simulink model "model_V2slx"  (R2024b)
settings: Solver=VariableStepAuto  StartTime=0.0  StopTime=30  RelTol=1e-3
values from neighbouring files (symbols this model uses):
  L = Simulink.Parameter    [initialization.m]    (also in mpc_v2.m = 0.35)
  Ts = 0.02    [mpc_v2.m]
libraries: simulink_extras x3, drivingscenarioandsensors x2, mpclib x1, robotmobilelib x1
settings Model: Creator=zanhe  LastModifiedBy=zanhe
settings OptimizationCC: DefaultParameterBehavior=Inlined  UseDivisionForNetSlopeComputation=on  GainParamInheritBuiltInType=on  UseFloatMulNetSlope=on  InlineInvariantSignals=on  PassReuseOutputArgsAs=Individual arguments  ZeroExternalMemoryAtStartup=off  ZeroInternalMemoryAtStartup=off  NoFixptDivByZeroProtection=on  EfficientFloat2IntCast=on  LifeSpan=1  OptimizeBlockOrder=speed  DifferentSizesBufferReuse=on  EfficientTunableParamExpr=on
settings DebuggingCC: ParameterTunabilityLossMsg=error  UniqueDataStoreMsg=error
settings HardwareCC: ProdBitPerPointer=32  ProdBitPerSizeT=32  ProdBitPerPtrDiffT=32  ProdLargestAtomicInteger=Long  ProdLargestAtomicFloat=Double  ProdWordSize=32  ProdLongLongMode=on  ProdHWDeviceType=ARM Compatible->ARM Cortex-M
settings SFSimCC: MATLABDynamicMemAlloc=off
settings RTWCC: Description=Embedded Coder  SystemTargetFile=ert.tlc  TemplateMakefile=ert_default_tmf
settings CodeAppCC: ForceParamTrailComments=on  IgnoreCustomStorageClasses=off  OperatorAnnotations=on  SimulinkDataObjDesc=on  SFDataObjDesc=on  CustomSymbolStrGlobalVar=rt$N$M  CustomSymbolStrType=$N$M  CustomSymbolStrFcn=$N$M$F  CustomSymbolStrMacro=$N$M  InsertBlockDesc=on
settings ERTTargetCC: TargetLangStandard=C99 (ISO)  GenerateSampleERTMain=on  IncludeMdlTerminateFcn=off  CombineSignalStateStructs=on  SupportAbsoluteTime=off  SupportComplex=off  SupportNonInlinedSFcns=on  ERTCustomFileTemplate=example_file_process.tlc  ERTFilePackagingFormat=CompactWithDataFile

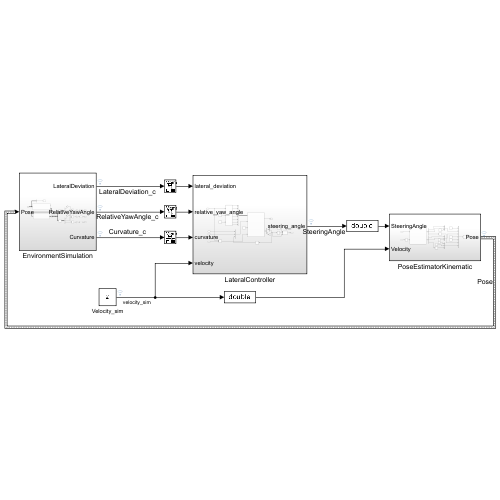
[thumbnail: Simulink's stored preview of the top-level diagram]
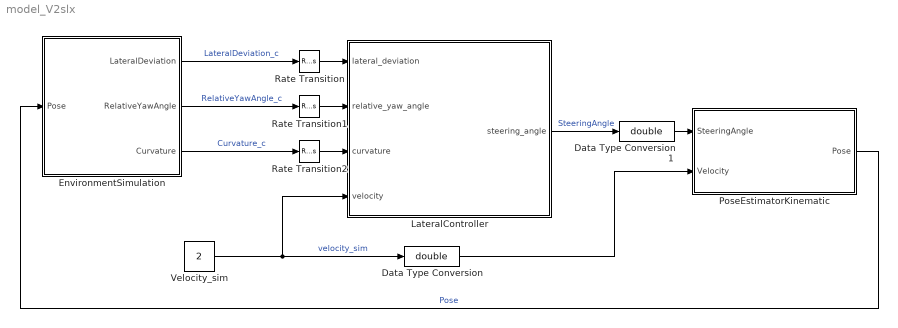
== system model_V2slx ==
  Data Type Conversion : DataTypeConversion  OutDataTypeStr=double  SaturateOnIntegerOverflow=off  RndMeth=Floor
  Data Type Conversion1 : DataTypeConversion  OutDataTypeStr=double  SaturateOnIntegerOverflow=off  RndMeth=Floor
  EnvironmentSimulation : Subsystem
  LateralController : Subsystem
  PoseEstimatorKinematic : Subsystem
  Rate Transition : RateTransition  Deterministic=off  OutPortSampleTime=Ts
  Rate Transition1 : RateTransition  Deterministic=off  OutPortSampleTime=Ts
  Rate Transition2 : RateTransition  Deterministic=off  OutPortSampleTime=Ts
  Velocity_sim : Constant  Value=2  OutDataTypeStr=single
  wires:
  Rate Transition/1 -> LateralController/1(lateral_deviation)
  Data Type Conversion1/1 -> PoseEstimatorKinematic/1(SteeringAngle)
  EnvironmentSimulation/3(Curvature) -> Rate Transition2/1  "Curvature_c"
  Rate Transition1/1 -> LateralController/2(relative_yaw_angle)
  Rate Transition2/1 -> LateralController/3(curvature)
  Velocity_sim/1 -> LateralController/4(velocity), Data Type Conversion/1  "velocity_sim"
  EnvironmentSimulation/2(RelativeYawAngle) -> Rate Transition1/1  "RelativeYawAngle_c"
  Data Type Conversion/1 -> PoseEstimatorKinematic/2(Velocity)
  PoseEstimatorKinematic/1(Pose) -> EnvironmentSimulation/1(Pose)  "Pose"
  EnvironmentSimulation/1(LateralDeviation) -> Rate Transition/1  "LateralDeviation_c"
  LateralController/1(steering_angle) -> Data Type Conversion1/1  "SteeringAngle"

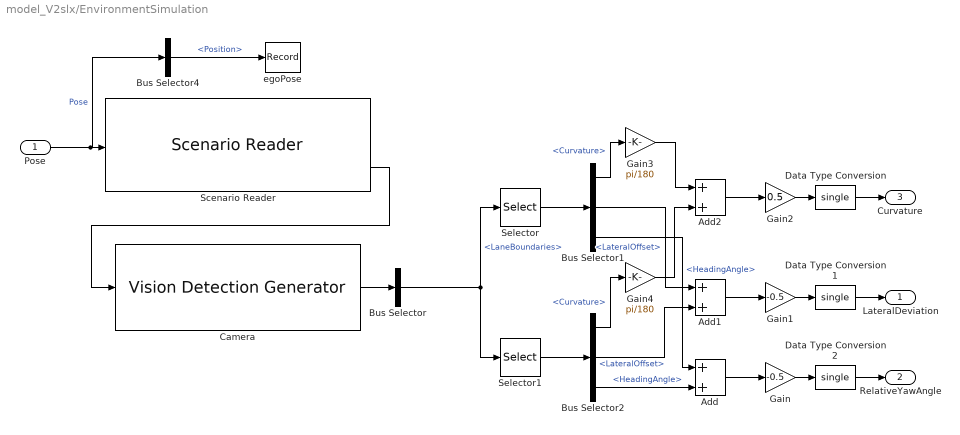
== system model_V2slx/EnvironmentSimulation ==
  Pose : Inport
  Add : Sum
  Add1 : Sum
  Add2 : Sum
  Bus Selector : BusSelector  OutputSignals=LaneBoundaries
  Bus Selector1 : BusSelector  OutputSignals=Curvature,LateralOffset,HeadingAngle
  Bus Selector2 : BusSelector  OutputSignals=Curvature,LateralOffset,HeadingAngle
  Bus Selector4 : BusSelector  OutputSignals=Position
  Camera : drivingscenarioandsensors/Vision Detection Generator  SensorIndex=1  DetectorOutput=Lanes only  UpdateInterval=0.05  LaneUpdateInterval=0.05  SensorLocation=[0.15 0]  Height=0.25  Yaw=0  Pitch=-10  Roll=0  BusNameSource=Auto  BusName=BusObjectDetections  BusName2Source=Auto  BusName2=BusLaneDetections  MaxNumDetectionsSource=Property  MaxNumDetections=50  MaxNumLanesSource=Property  MaxNumLanes=2  DetectionCoordinates=Ego Cartesian  SimulateUsing=Interpreted execution  MaxRange=5  BoundingBoxAccuracy=5  ProcessNoiseIntensity=5  MaxSpeed=100  MaxAllowedOcclusion=0.5  MinObjectImageSize=[15 15]  DetectionProbability=0.9  FalsePositivesPerImage=0.1  MinLaneImageSize=[20 3]  LaneBoundaryAccuracy=3  HasNoise=on  InitialSeedSource=Repeatable  InitialSeed=0  UsedSeed=0  ActorProfilesSource=From Scenario Reader block  ActorProfilesParameters=driving.internal.ActorProfilesParameters  ActorProfilesExpression=[struct('ActorID',1,'ClassID',1,'Length',0.5,'Width',0.2,'Height',0.3,'OriginOffset',[-0.15 0 0],'MeshVertices',[0.4 0.1 0.183737024221453;0.4 -0.1 0.183737024221453;0.4 -0.1 0.0674740484429066;0.4 0.1 0.0674740484429066;0.4 0.1 0.183737024221453;0.275 0.1 0.21280276816609;0.275 -0.1 0.21280276816609;0.4 -0.1 0.183737024221453;0.2 0.08 0.3;0.05 0.08 0.3;0.05 -0.08 0.3;0.2 -0.08 0.3;-0.025 0.1 0.21280276816609;-0.1 0.1 0.183737024221453;-0.1 -0.1 0.183737024221453;-0.025 -0.1 0.21280276816609;0.4 0.1 0.183737024221453;0.4 0.1 0.0674740484429066;0.275 0.1 0.0674740484429066;0.275 0.1 0.21280276816609;0.275 0.1 0.21280276816609;0.275 0.1 0.0674740484429066;-0.025 0.1 0.0674740484429066;-0.025 0.1 0.21280276816609;-0.025 0.1 0.21280276816609;-0.025 0.1 0.0674740484429066;-0.1 0.1 0.0761937716262976;-0.1 0.1 0.183737024221453;0.275 0.1 0.21280276816609;-0.025 0.1 0.21280276816609;0.05 0.08 0.3;0.2 0.08 0.3;0.4 -0.1 0.183737024221453;0.4 -0.1 0.0674740484429066;0.275 -0.1 0.0674740484429066;0.275 -0.1 0.21280276816609;0.275 -0.1 0.21280276816609;0.275 -0.1 0.0674740484429066;-0.025 -0.1 0.0674740484429066;-0.025 -0.1 0.21280276816609;-0.025 -0.1 0.21280276816609;-0.025 -0.1 0.0674740484429066;-0.1 -0.1 0.0761937716262976;-0.1 -0.1 0.183737024221453;0.275 -0.1 0.21280276816609;-0.025 -0.1 0.21280276816609;0.05 -0.08 0.3;0.2 -0.08 0.3;-0.025 0.1 0.21280276816609;-0.025 -0.1 0.21280276816609;0.05 -0.08 0.3;0.05 0.08 0.3;0.275 -0.1 0.21280276816609;0.2 -0.08 0.3;0.2 0.08 0.3;0.275 0.1 0.21280276816609;-0.1 0.1 0.183737024221453;-0.1 0.1 0.0761937716262976;-0.1 -0.1 0.0761937716262976;-0.1 -0.1 0.183737024221453;0.4 0.1 0.0674740484429066;0.4 -0.1 0.0674740484429066;-0.025 -0.1 0.0674740484429066;-0.025 0.1 0.0674740484429066;-0.025 0.1 0.0674740484429066;-0.1 0.1 0.0761937716262976;-0.1 -0.1 0.0761937716262976;-0.025 -0.1 0.0674740484429066;0.00638297872340421 -0.07 0;0.00638297872340421 -0.0966666666666667 0;0.0267053411696865 -0.07 0.0128863965733167;0.0267053411696865 -0.0966666666666667 0.0128863965733167;0.0392652518931835 -0.07 0.04662342079477;0.0392652518931835 -0.0966666666666667 0.04662342079477;0.0392652518931835 -0.07 0.0883246760910432;0.0392652518931835 -0.0966666666666667 0.0883246760910432;0.0267053411696865 -0.07 0.122061700312496;0.0267053411696865 -0.0966666666666667 0.122061700312496;0.00638297872340421 -0.07 0.134948096885813;0.00638297872340421 -0.0966666666666667 0.134948096885813;-0.0139393837228781 -0.07 0.122061700312496;-0.0139393837228781 -0.0966666666666667 0.122061700312496;-0.026499294446375 -0.07 0.0883246760910432;-0.026499294446375 -0.0966666666666667 0.0883246760910432;-0.026499294446375 -0.07 0.04662342079477;-0.026499294446375 -0.0966666666666667 0.04662342079477;-0.0139393837228781 -0.07 0.0128863965733167;-0.0139393837228781 -0.0966666666666667 0.0128863965733167;0.00638297872340421 -0.07 0;0.00638297872340421 -0.0966666666666667 0;0.00638297872340421 -0.07 0;0.0267053411696865 -0.07 0.0128863965733167;0.0392652518931835 -0.07 0.04662342079477;0.0392652518931835 -0.07 0.0883246760910432;0.0267053411696865 -0.07 0.122061700312496;0.00638297872340421 -0.07 0.134948096885813;-0.0139393837228781 -0.07 0.122061700312496;-0.026499294446375 -0.07 0.0883246760910432;-0.026499294446375 -0.07 0.04662342079477;-0.0139393837228781 -0.07 0.0128863965733167;0.00638297872340421 -0.0966666666666667 0;0.0267053411696865 -0.0966666666666667 0.0128863965733167;0.0392652518931835 -0.0966666666666667 0.04662342079477;0.0392652518931835 -0.0966666666666667 0.0883246760910432;0.0267053411696865 -0.0966666666666667 0.122061700312496;0.00638297872340421 -0.0966666666666667 0.134948096885813;-0.0139393837228781 -0.0966666666666667 0.122061700312496;-0.026499294446375 -0.0966666666666667 0.0883246760910432;-0.026499294446375 -0.0966666666666667 0.04662342079477;-0.0139393837228781 -0.0966666666666667 0.0128863965733167;0.00638297872340421 0.0966666666666667 0;0.00638297872340421 0.07 0;0.0267053411696865 0.0966666666666667 0.0128863965733167;0.0267053411696865 0.07 0.0128863965733167;0.0392652518931835 0.0966666666666667 ...(+5680 chars)],'MeshFaces',[1 2 3;3 4 1;5 6 7;7 8 5;9 10 11;11 12 9;13 14 15;15 16 13;17 18 19;19 20 17;21 22 23;23 24 21;25 26 27;27 28 25;29 30 31;31 32 29;33 34 35;35 36 33;37 38 39;39 40 37;41 42 43;43 44 41;45 46 47;47 48 45;49 50 51;51 52 49;53 54 55;55 56 53;57 58 59;59 60 57;61 62 63;63 64 61;65 66 67;67 68 65;69 71 72;72 70 69;71 73 74;74 72 71;73 75 76;76 74 73;75 77 78;78 76 75;77 79 80;80 78 77;79 81 82;82 80 79;81 83 84;84 82 81;83 85 86;86 84 83;85 87 88;88 86 85;87 89 90;90 88 87;91 92 93;91 93 94;91 94 95;91 95 96;91 96 97;91 97 98;91 98 99;91 99 100;101 102 103;101 103 104;101 104 105;101 105 106;101 106 107;101 107 108;101 108 109;101 109 110;111 113 114;114 112 111;113 115 116;116 114 113;115 117 118;118 116 115;117 119 120;120 118 117;119 121 122;122 120 119;121 123 124;124 122 121;123 125 126;126 124 123;125 127 128;128 126 125;127 129 130;130 128 127;129 131 132;132 130 129;133 134 135;133 135 136;133 136 137;133 137 138;133 138 139;133 139 140;133 140 141;133 141 142;143 144 145;143 145 146;143 146 147;143 147 148;143 148 149;143 149 150;143 150 151;143 151 152;153 155 156;156 154 153;155 157 158;158 156 155;157 159 160;160 158 157;159 161 162;162 160 159;161 163 164;164 162 161;163 165 166;166 164 163;165 167 168;168 166 165;167 169 170;170 168 167;169 171 172;172 170 169;171 173 174;174 172 171;175 176 177;175 177 178;175 178 179;175 179 180;175 180 181;175 181 182;175 182 183;175 183 184;185 186 187;185 187 188;185 188 189;185 189 190;185 190 191;185 191 192;185 192 193;185 193 194;195 197 198;198 196 195;197 199 200;200 198 197;199 201 202;202 200 199;201 203 204;204 202 201;203 205 206;206 204 203;205 207 208;208 206 205;207 209 210;210 208 207;209 211 212;212 210 209;211 213 214;214 212 211;213 215 216;216 214 213;217 218 219;217 219 220;217 220 221;217 221 222;217 222 223;217 223 224;217 224 225;217 225 226;227 228 229;227 229 230;227 230 231;227 231 232;227 232 233;227 233 234;227 234 235;227 235 236],'RCSPattern',[10 10;10 10],'RCSAzimuthAngles',[-180 180],'RCSElevationAngles',[-90 90])]  Intrinsics=driving.internal.cameraIntrinsics(FocalLength=[800 800],PrincipalPoint=[320 240],ImageSize=[580 740],RadialDistortion=[0 0],TangentialDistortion=[0 0],Skew=0)
  Data Type Conversion : DataTypeConversion  OutDataTypeStr=single  SaturateOnIntegerOverflow=off  RndMeth=Floor
  Data Type Conversion1 : DataTypeConversion  OutDataTypeStr=single  SaturateOnIntegerOverflow=off  RndMeth=Floor
  Data Type Conversion2 : DataTypeConversion  OutDataTypeStr=single  SaturateOnIntegerOverflow=off  RndMeth=Floor
  Gain : Gain  Gain=-0.5
  Gain1 : Gain  Gain=-0.5
  Gain2 : Gain  Gain=0.5
  Gain3 : Gain  Gain=pi/180
  Gain4 : Gain  Gain=pi/180
  Scenario Reader : drivingscenarioandsensors/Scenario Reader  ScenarioSource=From file  ScenarioFileName=C:\Users\zanhe\Documents\lateralVehicleController\SimulationModel\driving_scenarios\little_less_complex.mat  ScenarioVariableName=scenario  OutputCoordinateSystem=Vehicle coordinates  EgoVehicleSource=Input port  EgoVehicleActorID=1  OrientVehiclesOnRoad=off  OutputEgoVehiclePose=off  OutputEgoVehicleState=off  SampleTime=0.05  LaneBoundaryOutput=Ego vehicle lane boundaries  LaneBoundaryDistance=linspace(-20, 20, 101)  LaneBoundaryLocation=Center of lane markings  BusNameSource=Auto  BusName=BusActors  BusNumActorsSource=Scenario  BusNumActors=100  BusName2Source=Auto  BusName2=BusLaneBoundaries  BusNumLaneBoundariesSource=Scenario  BusNumLaneBoundaries=10  BusName3Source=Auto  BusName3=BusEgoActor  BusName4Source=Auto  BusName4=BusEgoState  ShowCoordinateLabels=on  SimulateUsing=Interpreted execution
  Selector : Selector  InputPortWidth=2  IndexOptions=Index vector (dialog)  Indices=1  OutputSizes=1
  Selector1 : Selector  InputPortWidth=2  IndexOptions=Index vector (dialog)  Indices=2  OutputSizes=1
  egoPose : Record  VariableName=egoPose  Filename=C:\Users\zanhe\Documents\lateralVehicleController\SimulationModel\SimulatedScenarios\path.mat  RecordToWorkspace=on  FileSettingsInternal="{\"entries\":[{\"content\":{\"excelSettings\":{\"content\":{},\"type\":\"Streamout.ExcelSettings\"}},\"type\":\"Streamout.FileSettingStorage\",\"uuid\":\"\"}],\"packageUris\":[\"http:\\/\\/schema.mathworks.com\\/mf0\\/streamout_blocks\\/R2020a\"],\"version\":\"1.0\"}"  Layout=[1 1]  SignalsInternal="{\"entries\":[{\"content\":{\"signals\":[{\"content\":{\"blockPath\":[],\"dimensions\":[1,3],\"domain\":\"\",\"hasChildren\":true,\"lineColor\":\"#ff6929\",\"lineWidth\":2,\"port\":1,\"signalID\":1,\"signalName\":\"<Position>\"},\"type\":\"RecordBlkView.Signal\",\"uuid\":\"\"},{\"content\":{\"blockPath\":[],\"channel\":[1,1],\"dimensions\":[1,3],\"domain\":\"\",\"lineColor\":\"#b746ff\",\"lineWidth\":2,\"parentID\":1,\"plots\":[ 1 ],\"port\":1,\"signalID\":2,\"signalName\":\"<Position>\"},\"type\":\"RecordBlkView.Signal\",\"uuid\":\"\"},{\"content\":{\"blockPath\":[],\"channel\":[1,2],\"dimensions\":[1,3],\"domain\":\"\",\"lineColor\":\"#edb120\",\"lineWidth\":2,\"parentID\":1,\"plots\":[ 1 ],\"port\":1,\"signalID\":3,\"signalName\":\"<Position>\"},\"type\":\"RecordBlkView.Signal\",\"uuid\":\"\"},{\"content\":{\"blockPath\":[],\"channel\":[1,3],\"dimensions\":[1,3],\"domain\":\"\",\"lineColor\":\"#7e2f8e\",\"lineWidth\":2,\"parentID\":1,\"plots\":[ 1 ],\"port\":1,\"signalID\":4,\"signalName\":\"<Position>\"},\"type\":\"RecordBlkView.Signal\",\"uuid\":\"\"}]},\"type\":\"RecordBlkView.InputSignals\",\"uuid\":\"\"}],\"packageUris\":[\"http:\\/\\/schema.mathworks.com\\/mf0\\/streamout_blocks\\/R2020a\"],\"version\":\"1.0\"}"  VisualizationBindings="{\"sparklinesplugin\":{\"info\":[{\"bindingParametersList\":[],\"subplotID\":1}]}}"
  LateralDeviation : Outport
  RelativeYawAngle : Outport  Port=2
  Curvature : Outport  Port=3
  wires:
  Pose/1 -> Bus Selector4/1, Scenario Reader/1  "Pose"
  Bus Selector1/3 -> Add/1  "<HeadingAngle>"
  Bus Selector2/3 -> Add/2  "<HeadingAngle>"
  Add/1 -> Gain/1
  Gain/1 -> Data Type Conversion2/1
  Add1/1 -> Gain1/1
  Add2/1 -> Gain2/1
  Bus Selector1/2 -> Add1/1  "<LateralOffset>"
  Bus Selector2/2 -> Add1/2  "<LateralOffset>"
  Bus Selector1/1 -> Gain3/1  "<Curvature>"
  Bus Selector2/1 -> Gain4/1  "<Curvature>"
  Gain1/1 -> Data Type Conversion1/1
  Gain2/1 -> Data Type Conversion/1
  Selector/1 -> Bus Selector1/1
  Bus Selector/1 -> Selector/1, Selector1/1  "<LaneBoundaries>"
  Selector1/1 -> Bus Selector2/1
  Data Type Conversion/1 -> Curvature/1
  Camera/1 -> Bus Selector/1
  Scenario Reader/2 -> Camera/1
  Data Type Conversion1/1 -> LateralDeviation/1
  Data Type Conversion2/1 -> RelativeYawAngle/1
  Bus Selector4/1 -> egoPose/1  "<Position>"
  Gain3/1 -> Add2/1
  Gain4/1 -> Add2/2

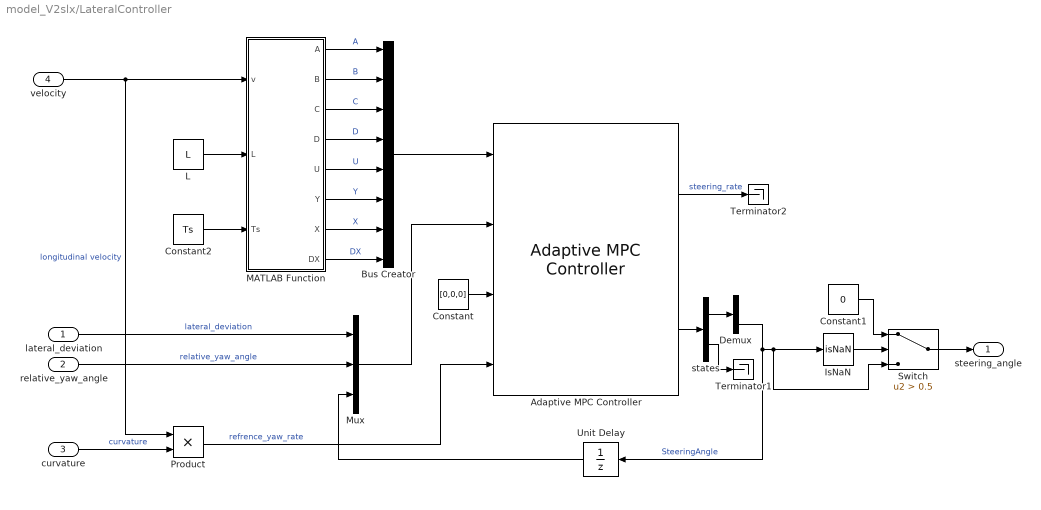
== system model_V2slx/LateralController ==
  lateral_deviation : Inport  OutDataTypeStr=single
  relative_yaw_angle : Inport  Port=2  OutDataTypeStr=single
  curvature : Inport  Port=3  OutDataTypeStr=single
  velocity : Inport  Port=4  OutDataTypeStr=single
  Adaptive MPC Controller : mpclib/Adaptive MPC Controller  SCDEnableBlockLinearizationSpecification=on  mpcobj=mpc1  enable_value=0  updateMPCinCallerWorkspace=on  md_inport=on  mv_inport=off  uref_inport=off  return_cost=off  return_mvseq=off  return_qpstatus=off  return_xseq=off  return_state=on  return_ovseq=off  state_inport=off  isltv_plant=off  umin_inport=off  umax_inport=off  ymin_inport=off  ymax_inport=off  cc_inport=off  ywt_inport=off  uwt_inport=off  duwt_inport=off  rhoeps_inport=off  pm_inport=off  MaximumP=10  HorizonChoice=FixedHorizon  BlockDataType=single  SampleTimeInherited=off  switch_inport=off
  Bus Creator : BusCreator  Inputs=8
  Constant : Constant  Value=[0,0,0]  OutDataTypeStr=single
  Constant1 : Constant  Value=0  OutDataTypeStr=single
  Constant2 : Constant  Value=Ts
  Demux : Demux  Outputs=3
  IsNaN : RelationalOperator  Operator=isNaN  OutDataTypeStr=boolean  RndMeth=Simplest  InputSameDT=off
  L : Constant  Value=L
  MATLAB Function : MATLAB Function  TreatAsAtomicUnit=on
  Mux : Mux  Inputs=3
  Product : Product  OutDataTypeStr=single
  Switch : Switch  Criteria=u2 > Threshold  Threshold=0.5  OutDataTypeStr=single  SaturateOnIntegerOverflow=off  InputSameDT=off
  Terminator1 : Terminator
  Terminator2 : Terminator
  Unit Delay : UnitDelay  SampleTime=-1  HasFrameUpgradeWarning=on
  states : Demux  Outputs=2
  steering_angle : Outport  OutDataTypeStr=single
  wires:
  MATLAB Function/5(U) -> Bus Creator/5  "U"
  MATLAB Function/4(D) -> Bus Creator/4  "D"
  MATLAB Function/6(Y) -> Bus Creator/6  "Y"
  MATLAB Function/7(X) -> Bus Creator/7  "X"
  MATLAB Function/1(A) -> Bus Creator/1  "A"
  MATLAB Function/3(C) -> Bus Creator/3  "C"
  MATLAB Function/8(DX) -> Bus Creator/8  "DX"
  MATLAB Function/2(B) -> Bus Creator/2  "B"
  Bus Creator/1 -> Adaptive MPC Controller/1
  L/1 -> MATLAB Function/2(L)
  velocity/1 -> Product/1, MATLAB Function/1(v)  "longitudinal velocity"
  Constant/1 -> Adaptive MPC Controller/3
  lateral_deviation/1 -> Mux/1  "lateral_deviation"
  relative_yaw_angle/1 -> Mux/2  "relative_yaw_angle"
  Mux/1 -> Adaptive MPC Controller/2
  curvature/1 -> Product/2  "curvature"
  Product/1 -> Adaptive MPC Controller/4  "refrence_yaw_rate"
  IsNaN/1 -> Switch/2
  Constant1/1 -> Switch/1
  Switch/1 -> steering_angle/1
  Constant2/1 -> MATLAB Function/3(Ts)
  Adaptive MPC Controller/2 -> states/1
  states/2 -> Terminator1/1
  states/1 -> Demux/1
  Demux/3 -> IsNaN/1, Switch/3, Unit Delay/1  "SteeringAngle"
  Unit Delay/1 -> Mux/3
  Adaptive MPC Controller/1 -> Terminator2/1  "steering_rate"

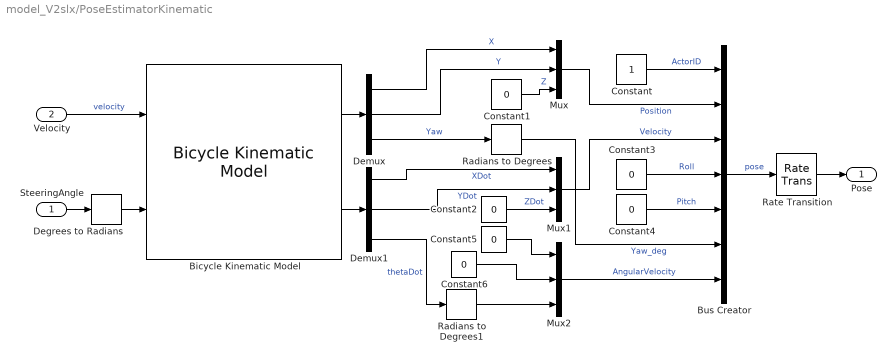
== system model_V2slx/PoseEstimatorKinematic ==
  SteeringAngle : Inport
  Velocity : Inport  Port=2
  Bicycle Kinematic Model : robotmobilelib/Bicycle Kinematic Model  VehicleInputs=Vehicle Speed & Steering Angle  WheelBase=0.35  VehicleSpeedRange=[-inf inf]  MaxSteeringAngle=pi/4  InitialState=[0; 0; 0]  SimulateUsing=Interpreted execution
  Bus Creator : BusCreator  Inputs=7  OutDataTypeStr=Bus: slBus1  NonVirtualBus=on
  Constant : Constant
  Constant{1..6} (6 alike) : Constant  Value=0
  Degrees to Radians : simulink_extras/Transformations/Degrees to Radians
  Demux : Demux  Outputs=3
  Demux1 : Demux  Outputs=3
  Mux : Mux  Inputs=3
  Mux1 : Mux  Inputs=3
  Mux2 : Mux  Inputs=3
  Radians to Degrees : simulink_extras/Transformations/Radians to Degrees
  Radians to Degrees1 : simulink_extras/Transformations/Radians to Degrees
  Rate Transition : RateTransition  OutPortSampleTimeOpt=Inherit
  Pose : Outport  OutDataTypeStr=Bus: slBus1
  wires:
  Bus Creator/1 -> Rate Transition/1  "pose"
  Velocity/1 -> Bicycle Kinematic Model/1  "velocity"
  SteeringAngle/1 -> Degrees to Radians/1
  Bicycle Kinematic Model/1 -> Demux/1
  Demux/1 -> Mux/1  "X"
  Demux/2 -> Mux/2  "Y"
  Bicycle Kinematic Model/2 -> Demux1/1
  Demux1/1 -> Mux1/1  "XDot"
  Demux1/2 -> Mux1/2  "YDot"
  Demux1/3 -> Radians to Degrees1/1  "thetaDot"
  Constant/1 -> Bus Creator/1  "ActorID"
  Mux/1 -> Bus Creator/2  "Position"
  Constant1/1 -> Mux/3  "Z"
  Constant2/1 -> Mux1/3  "ZDot"
  Mux1/1 -> Bus Creator/3  "Velocity"
  Constant3/1 -> Bus Creator/4  "Roll"
  Constant4/1 -> Bus Creator/5  "Pitch"
  Demux/3 -> Radians to Degrees/1  "Yaw"
  Constant5/1 -> Mux2/1
  Constant6/1 -> Mux2/2
  Mux2/1 -> Bus Creator/7  "AngularVelocity"
  Rate Transition/1 -> Pose/1
  Radians to Degrees/1 -> Bus Creator/6  "Yaw_deg"
  Radians to Degrees1/1 -> Mux2/3
  Degrees to Radians/1 -> Bicycle Kinematic Model/2

== matlab function model_V2slx/LateralController/MATLAB Function ==
  data: v input; A output; L input; B output; C output; D output; U output; Y output; X output; DX output; Ts input
function [A, B, C ,D, U, Y, X, DX]= fcn(v, L, Ts)

Ac = [0  v v;
     0  0 v/L;
     0  0  0];

Bc = [0 0;
     0 -1;
     1 0];


C = [1 0 0;
     0 1 0;
     0 0 1];
D = [0 0;
     0 0;
     0 0];

% Discretize the continus A and B matricies
n = size(Ac, 1);
m = size(Bc, 2);

M = [Ac Bc;
    zeros(m, n+m)];

M_exp = expm(M*Ts);

A = M_exp(1:n, 1:n);
B = M_exp(1:n, n+1:n+m);

X = zeros(3, 1);
U = zeros(2, 1);
Y = zeros(3, 1);
DX = zeros(3, 1);
